simulink model "Boeing787_Yue"  (R2013a)
settings: Solver=ode23tb  SolverMode=SingleTasking  StartTime=0.0  StopTime=346  RelTol=1e-3
InitFcn:
  | load('SampleOutput.mat')
  | 
  | load('SampleFuelBurn.mat')
values from neighbouring files (symbols this model uses):
  FuelBurn = [0 0 0 0 0 0 0 0 0 0 0 0 ... (18249 elements, 1x18249)]    [Benchmark_data1.mat]
undefined symbols (not defined in the file or in its folder): ailerons, AirProp, B_737, elevator, HydProp, landing_gear, rudder, thrust_rev
libraries: PowerFlowLib x118, simulink x20
(part 1 of 26)
settings Model: Creator=Bradford  LastModifiedBy=caoyue
settings DataIOCC: SignalLoggingSaveFormat=ModelDataLogs
settings OptimizationCC: BlockReduction=off  BooleanDataType=off
settings DebuggingCC: SaveWithParameterizedLinksMsg=none  SignalResolutionControl=TryResolveAllWithWarning  SolverPrmCheckMsg=none  MultiTaskDSMMsg=warning  MultiTaskCondExecSysMsg=none  StrictBusMsg=None
settings HardwareCC: TargetUnknown=on
settings RTWCC: IncludeERTFirstTime=on
settings GRTTargetCC: CodeReplacementLibrary=None  CPPClassGenCompliant=on

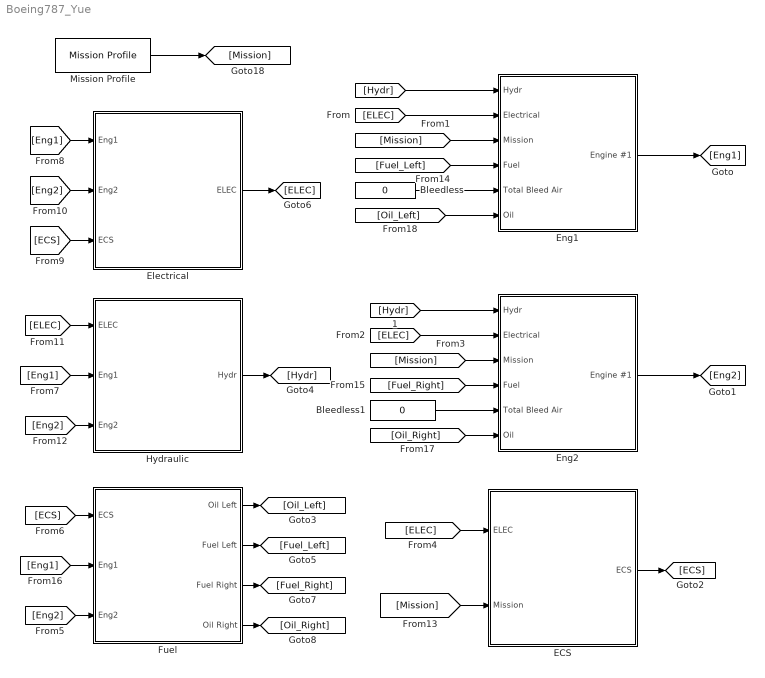
== system Boeing787_Yue ==
  Bleedless : Constant  Value=0
  Bleedless1 : Constant  Value=0
  ECS : Subsystem
  Electrical : Subsystem
  Eng1 : Subsystem
  Eng2 : Subsystem
  Fuel : Subsystem
  Hydraulic : Subsystem
  Mission Profile : PowerFlowLib/Mission Profile/Mission Profile  mssn_check=off  mssn_prof=MSSN  del_P=0  del_T=0  del_rho=0  pres_msl=101.3  temp_msl=15  dens_msl=1.229
  wires:
  [ELEC] -> Eng1/2(Electrical)
  [Mission] -> Eng1/3(Mission)
  [Hydr] -> Eng1/1(Hydr)
  Eng1/1(Engine #1) -> [Eng1]
  [ELEC] -> ECS/1(ELEC)
  ECS/1(ECS) -> [ECS]
  [ECS] -> Fuel/1(ECS)
  Fuel/1(Oil Left) -> [Oil_Left]
  [Eng1] -> Hydraulic/2(Eng1)
  Hydraulic/1("Hydr ") -> [Hydr]
  [Eng1] -> Electrical/1(Eng1)
  [ECS] -> Electrical/3(ECS)
  Mission Profile/1 -> [Mission]
  [Eng2] -> Electrical/2(Eng2)
  Electrical/1(ELEC) -> [ELEC]
  [ELEC] -> Hydraulic/1(ELEC)
  [Eng2] -> Hydraulic/3(Eng2)
  [Mission] -> ECS/2(Mission)
  Bleedless/1 -> Eng1/5(Total Bleed Air)
  [Eng1] -> Fuel/2(Eng1)
  [Eng2] -> Fuel/3(Eng2)
  [Fuel_Left] -> Eng1/4(Fuel)
  Fuel/2(Fuel Left) -> [Fuel_Left]
  Fuel/3(Fuel Right) -> [Fuel_Right]
  Fuel/4(Oil Right) -> [Oil_Right]
  [Oil_Left] -> Eng1/6(Oil)
  [ELEC] -> Eng2/2(Electrical)
  [Mission] -> Eng2/3(Mission)
  [Hydr] -> Eng2/1(Hydr)
  Eng2/1(Engine #1) -> [Eng2]
  Bleedless1/1 -> Eng2/5(Total Bleed Air)
  [Fuel_Right] -> Eng2/4(Fuel)
  [Oil_Right] -> Eng2/6(Oil)

== system Boeing787_Yue/ECS ==
  ELEC : Inport
  Mission : Inport  Port=2
  Bus Selector : BusSelector  OutputSignals=Flight parameters
  Bus Selector1 : BusSelector  OutputSignals=DC_Voltage_270
  Bus Selector2 : BusSelector  OutputSignals=temp_K,Mach
  Bus Selector3 : BusSelector  OutputSignals=power_kW
  Cabin Zone1 : PowerFlowLib/Energy & Power Systems/Thermal/ECS/Cabin Zone  A_fuselage=880  V_cab=245  n_pass=300  L_shell=0.003  K_shell=1  L_insulation=0.02  K_insulation=1  L_coating=0.002  K_coating=1  Vdot_sa_pass=0.009438  q_pass=60  RAR=.25  h_outside=1  h_inside=1
  Electrical Sink Cabin : Subsystem
  Fan2 : PowerFlowLib/Energy & Power Systems/Thermal/ECS/Fan  N_fan=1725
  Left Pack : Subsystem
  Memory : Memory
  Place holder : Constant
  Right Pack1 : Subsystem
  Scope : Scope
      settings: SaveName=ScopeData37
  Thermal Loads : Subsystem
  n-intlet Mixing Junction : PowerFlowLib/Energy & Power Systems/Thermal/ECS/n-intlet Mixing Junction  no_inlets=3  d_in_1=0.1  d_in_2=0.1  d_out=0.2
  ECS : Outport
  wires:
  Mission/1 -> Bus Selector/1
  ELEC/1 -> Bus Selector1/1
  Bus Selector/1 -> [Ambient_Cond]  "<Flight parameters>"
  Left Pack/1(Flow Out) -> n-intlet Mixing Junction/2
  Right Pack1/1(Flow Out) -> n-intlet Mixing Junction/3
  n-intlet Mixing Junction/1 -> [Second_HX_Flow], Memory/1
  Memory/1 -> Cabin Zone1/1
  [Ambient_Cond] -> Bus Selector2/1
  Bus Selector2/1 -> Cabin Zone1/2  "<temp_K>"
  Bus Selector2/2 -> Cabin Zone1/3  "<Mach>"
  Thermal Loads/1("Thermal Loads ") -> Cabin Zone1/4
  Cabin Zone1/2 -> Fan2/1
  Cabin Zone1/1 -> Scope/1, [Cabin_conditions]
  Fan2/2 -> Bus Selector3/1
  Bus Selector3/1 -> Electrical Sink Cabin/1(In1)  "<power_kW>"
  Fan2/1 -> [Fan_Mixing_Jn]
  [Fan_Mixing_Jn] -> n-intlet Mixing Junction/1
  [Voltage] -> Left Pack/1(Voltage)
  [Voltage] -> Right Pack1/1(Voltage)
  [Ambient_Cond] -> Left Pack/2(Ambient)
  [Ambient_Cond] -> Right Pack1/2(Ambient)
  Bus Selector1/1 -> [Voltage]  "<DC_Voltage_270>"
  Place holder/1 -> ECS/1
